simulink model "twsbr_lqi"  (R2026a)
settings: Solver=ode45  StopTime=8.0  MaxStep=0.001  RelTol=1e-9  AbsTol=1e-11
model workspace (MAT data in the model file):
  controller_reset_data = [0  1; 0.001  0; 8  0]
  disturbance_force_data = [0  0; 8  0]
  disturbance_torque_data = [0  0; 8  0]
  position_reference_data = [0  0; 8  0]
undefined symbols (not defined in the file): DiscIntNeverNeededParam
settings Model: Creator=Linxiuqi  LastModifiedBy=Linxiuqi

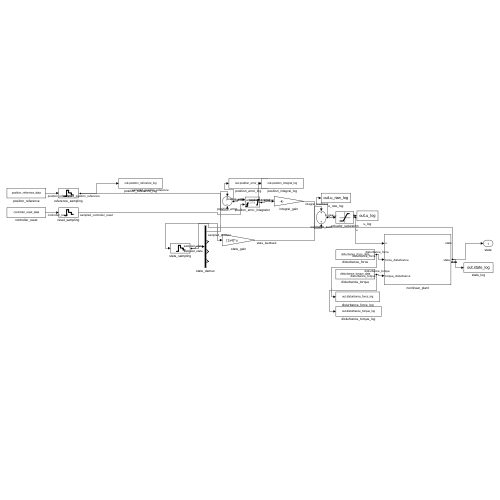
[thumbnail: Simulink's stored preview of the top-level diagram]
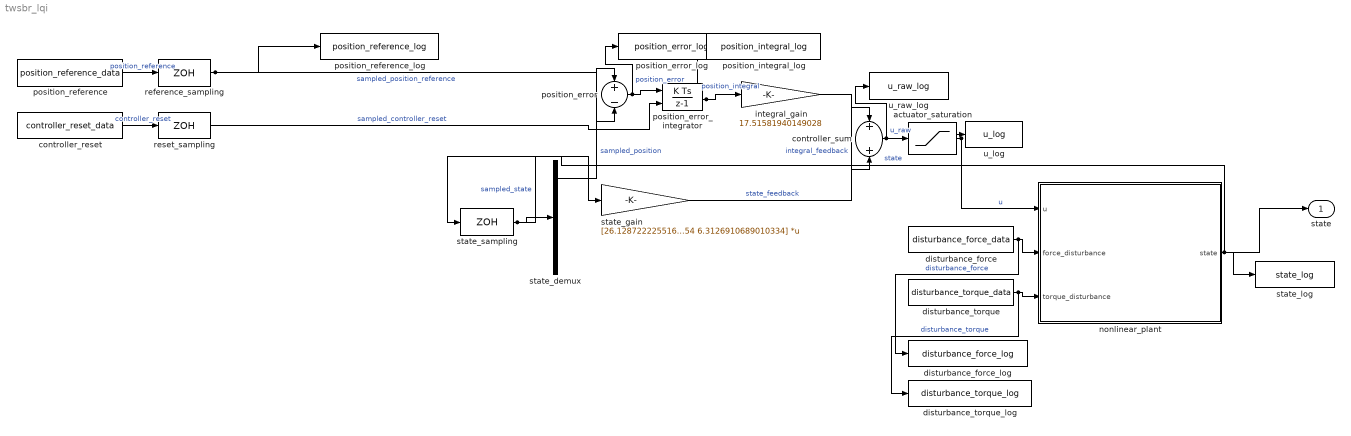
== system twsbr_lqi ==
  actuator_saturation : Saturate  UpperLimit=1  LowerLimit=-1
  controller_reset : FromWorkspace  VariableName=controller_reset_data  Interpolate=off  OutputAfterFinalValue=Holding final value
  controller_sum : Sum
  disturbance_force : FromWorkspace  VariableName=disturbance_force_data  Interpolate=off  OutputAfterFinalValue=Holding final value
  disturbance_force_log : ToWorkspace  VariableName=disturbance_force_log  SaveFormat=Structure With Time  SampleTime=-1
  disturbance_torque : FromWorkspace  VariableName=disturbance_torque_data  Interpolate=off  OutputAfterFinalValue=Holding final value
  disturbance_torque_log : ToWorkspace  VariableName=disturbance_torque_log  SaveFormat=Structure With Time  SampleTime=-1
  integral_gain : Gain  Gain=17.51581940149028
  nonlinear_plant : Subsystem
  position_error : Sum  Inputs=+-
  position_error_integrator : DiscreteIntegrator  gainval=1  ExternalReset=rising  InitialCondition=0.0  SampleTime=0.01  LimitOutput=on  UpperSaturationLimit=1000000  LowerSaturationLimit=-1000000  ICPrevOutput=DiscIntNeverNeededParam  ICPrevScaledInput=DiscIntNeverNeededParam
  position_error_log : ToWorkspace  VariableName=position_error_log  SaveFormat=Structure With Time  SampleTime=-1
  position_integral_log : ToWorkspace  VariableName=position_integral_log  SaveFormat=Structure With Time  SampleTime=-1
  position_reference : FromWorkspace  VariableName=position_reference_data  Interpolate=off  OutputAfterFinalValue=Holding final value
  position_reference_log : ToWorkspace  VariableName=position_reference_log  SaveFormat=Structure With Time  SampleTime=-1
  reference_sampling : ZeroOrderHold  SampleTime=0.01
  reset_sampling : ZeroOrderHold  SampleTime=0.01
  state_demux : Demux
  state_gain : Gain  Gain=[26.128722225516054 14.435345464225271 38.084885568122154 6.3126910689010334]  Multiplication=Matrix(K*u)
  state_log : ToWorkspace  VariableName=state_log  SaveFormat=Structure With Time  SampleTime=-1
  state_sampling : ZeroOrderHold  SampleTime=0.01
  u_log : ToWorkspace  VariableName=u_log  SaveFormat=Structure With Time  SampleTime=-1
  u_raw_log : ToWorkspace  VariableName=u_raw_log  SaveFormat=Structure With Time  SampleTime=-1
  state : Outport
  wires:
  position_reference/1 -> reference_sampling/1  "position_reference"
  reference_sampling/1 -> position_error/2, position_reference_log/1  "sampled_position_reference"
  controller_reset/1 -> reset_sampling/1  "controller_reset"
  reset_sampling/1 -> position_error_integrator/2  "sampled_controller_reset"
  nonlinear_plant/1(state) -> state_sampling/1, state/1, state_log/1  "state"
  state_sampling/1 -> state_demux/1, state_gain/1  "sampled_state"
  state_demux/1 -> position_error/1  "sampled_position"
  position_error/1 -> position_error_integrator/1, position_error_log/1  "position_error"
  position_error_integrator/1 -> integral_gain/1, position_integral_log/1  "position_integral"
  state_gain/1 -> controller_sum/1  "state_feedback"
  integral_gain/1 -> controller_sum/2  "integral_feedback"
  controller_sum/1 -> actuator_saturation/1, u_raw_log/1  "u_raw"
  actuator_saturation/1 -> nonlinear_plant/1(u), u_log/1  "u"
  disturbance_force/1 -> nonlinear_plant/2(force_disturbance), disturbance_force_log/1  "disturbance_force"
  disturbance_torque/1 -> nonlinear_plant/3(torque_disturbance), disturbance_torque_log/1  "disturbance_torque"

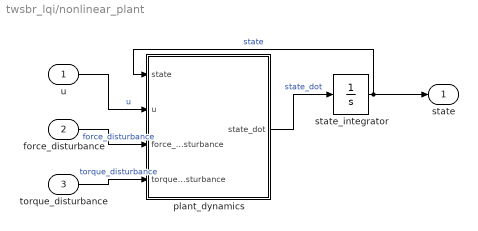
== system twsbr_lqi/nonlinear_plant ==
  u : Inport
  force_disturbance : Inport  Port=2
  torque_disturbance : Inport  Port=3
  plant_dynamics : MATLAB Function  TreatAsAtomicUnit=on
  state_integrator : Integrator  InitialCondition=[0;0;0;0]
  state : Outport
  wires:
  plant_dynamics/1(state_dot) -> state_integrator/1  "state_dot"
  torque_disturbance/1 -> plant_dynamics/4(torque_disturbance)  "torque_disturbance"
  force_disturbance/1 -> plant_dynamics/3(force_disturbance)  "force_disturbance"
  u/1 -> plant_dynamics/2(u)  "u"
  state_integrator/1 -> state/1, plant_dynamics/1(state)  "state"

== matlab function twsbr_lqi/nonlinear_plant/plant_dynamics ==
  data: state input; u input; state_dot output; force_disturbance input; torque_disturbance input
function state_dot = plant_dynamics(state, u, force_disturbance, torque_disturbance)
%#codegen
body_mass = 1.2;
wheel_mass = 0.29999999999999999;
com_length = 0.17999999999999999;
body_inertia = 0.025000000000000001;
damping = 0.050000000000000003;
gravity = 9.8100000000000005;
motor_gain = 12;
x_dot = state(2);
theta = state(3);
theta_dot = state(4);
force = motor_gain * u + force_disturbance;
mass_sum = wheel_mass + body_mass;
rotational_term = body_inertia + body_mass * com_length^2;
coupling = body_mass * com_length * cos(theta);
rhs_position = force - damping * x_dot + body_mass * com_length * theta_dot^2 * sin(theta);
rhs_angle = body_mass * gravity * com_length * sin(theta) + torque_disturbance;
determinant = mass_sum * rotational_term - coupling^2;
x_ddot = (rotational_term * rhs_position - coupling * rhs_angle) / determinant;
theta_ddot = (-coupling * rhs_position + mass_sum * rhs_angle) / determinant;
state_dot = [x_dot; x_ddot; theta_dot; theta_ddot];
end
